simulink model "homework2"  (R2018a)
settings: Solver=VariableStepAuto  StartTime=0.0  StopTime=30.0  RelTol=1e-5
settings Model: Creator=dell  LastModifiedBy=dell

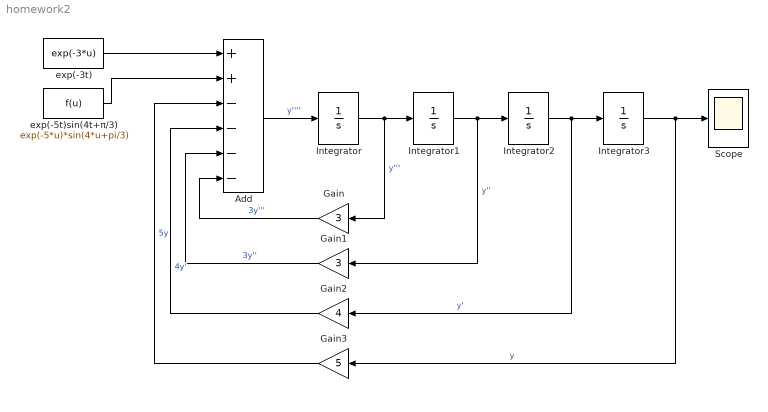
== system homework2 ==
  Add : Sum  Inputs=++----
  Gain : Gain  Gain=3
  Gain1 : Gain  Gain=3
  Gain2 : Gain  Gain=4
  Gain3 : Gain  Gain=5
  Integrator : Integrator  InitialCondition=0.2
  Integrator1 : Integrator  InitialCondition=0.5
  Integrator2 : Integrator  InitialCondition=0.5
  Integrator3 : Integrator  InitialCondition=1
  Scope : Scope
  exp(-3t) : Fcn  Expr=exp(-3*u)
  exp(-5t)sin(4t+π/3) : Fcn  Expr=exp(-5*u)*sin(4*u+pi/3)
  wires:
  exp(-3t)/1 -> Add/1
  exp(-5t)sin(4t+π/3)/1 -> Add/2
  Add/1 -> Integrator/1  "y''''"
  Integrator/1 -> Gain/1, Integrator1/1  "y'''"
  Gain/1 -> Add/6  "3y'''"
  Integrator1/1 -> Gain1/1, Integrator2/1  "y''"
  Gain1/1 -> Add/5  "3y''"
  Integrator2/1 -> Gain2/1, Integrator3/1  "y'"
  Gain2/1 -> Add/4  "4y'"
  Integrator3/1 -> Gain3/1, Scope/1  "y"
  Gain3/1 -> Add/3  "5y"
